simulink model "sampleModel1876"  (R2023a)
settings: Solver=VariableStepAuto  StartTime=0.0  StopTime=10.0  RelTol=1e-3
libraries: hdlsllib x5
settings Model: Creator=user1  LastModifiedBy=user1

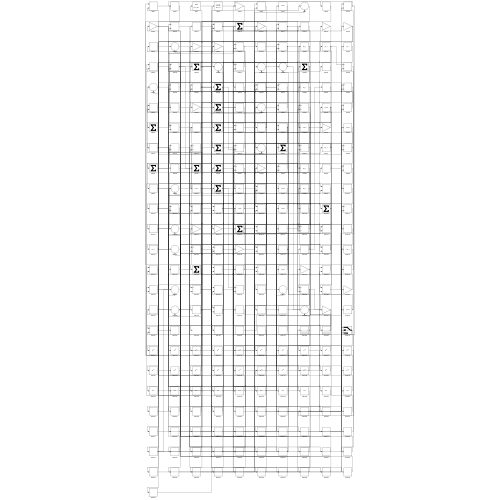
[thumbnail: Simulink's stored preview of the top-level diagram]
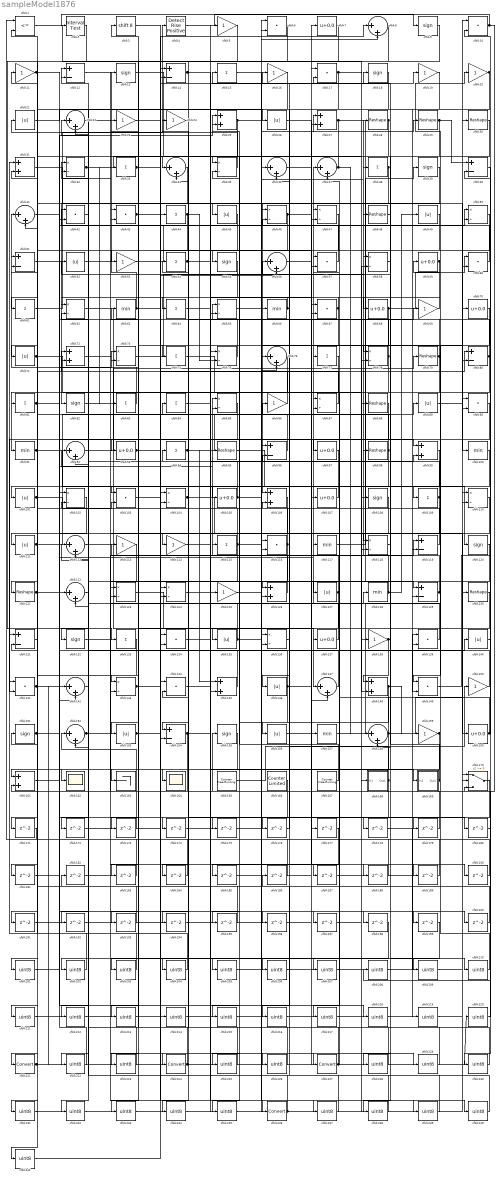
== system sampleModel1876 ==
  cfblk1 : RelationalOperator  Operator=<=  OutDataTypeStr=boolean  InputSameDT=off
  cfblk{6,10,17,42..43,57,60,67,90,103,116,134,139,141,144,149} (16 alike) : DotProduct  OutDataTypeStr=Inherit: Inherit via internal rule
  cfblk{63,66,91,100,117,128,157} (7 alike) : MinMax
  cfblk{21,26,45,49,52,71,89,101,111,127,135,140,146,153,156} (15 alike) : Abs  SaturateOnIntegerOverflow=off
  cfblk{32,35,46..47,50,58,62,65,73,75,78,85,87,102,104,110,118,123..124,136,143} (21 alike) : Product  Inputs=*/  RndMeth=Zero  SaturateOnIntegerOverflow=on
  cfblk{7,59,68,70,93,97,105,107,137,160} (10 alike) : Bias  Bias=0.0  SaturateOnIntegerOverflow=off
  cfblk{25,27,31,72,99,106,126,145,148,161} (10 alike) : Sum
  cfblk{9,13,18,39,55,82,108,120,132,151,155} (11 alike) : Signum
  cfblk{15,33,38,44,54,61,64,74,77,81,83..84,94,109,115,133} (16 alike) : Sum  Inputs=+
  cfblk{5,11,16,19..20,23..24,53,69,86,113..114,125,138,150,159} (16 alike) : Gain
  cfblk{8,22,34,36..37,41,56,76,92,112,122,142,147,152,158} (15 alike) : Sum  Inputs=|++
  cfblk{12,14,40,51,80,96,119,129,131,154} (10 alike) : Sum  Inputs=+-
  cfblk{28..30,48,79,88,95,98,121,130} (10 alike) : Reshape
  cfblk162 : Scope
  cfblk163 : Terminator
  cfblk164 : Scope
  cfblk165 : hdlsllib/Sources/Counter Free-Running  NumBits=16  tsamp=-1
  cfblk166 : hdlsllib/Sources/Counter Limited  uplimit=7  tsamp=-1
  cfblk167 : hdlsllib/Sources/Counter Free-Running  NumBits=16  tsamp=-1
  cfblk168 : Subsystem
      settings: LibrarySourceBlock=|
      | hdlsllib/Ports &
      | Subsystems/Subsystem
  cfblk169 : Subsystem
      settings: LibrarySourceBlock=|
      | hdlsllib/Ports &
      | Subsystems/Subsystem
  cfblk170 : Switch  SaturateOnIntegerOverflow=off  InputSameDT=off
  cfblk{171..200} (30 alike) : Delay  SampleTime=1
  cfblk2 : hdlsllib/Logic and Bit Operations/Interval Test  IntervalClosedRight=on  uplimit=0.5  IntervalClosedLeft=on  lowlimit=-0.5  OutDataTypeStr=boolean
  cfblk{201..220,222..223,225..226,228..235,237..241} (37 alike) : DataTypeConversion  OutDataTypeStr=uint8  SaturateOnIntegerOverflow=off  RndMeth=Floor
  cfblk{221,224,227,236} (4 alike) : DataTypeConversion  SaturateOnIntegerOverflow=off  RndMeth=Floor
  cfblk3 : ArithShift  BitShiftNumber=8
  cfblk4 : hdlsllib/Logic and Bit Operations/Detect Rise Positive  vinit=0  OutDataTypeStr=boolean
  wires:
  cfblk83/1 -> cfblk41/1
  cfblk47/1 -> cfblk153/1
  cfblk27/1 -> cfblk129/1, cfblk164/1, cfblk55/1
  cfblk2/1 -> cfblk133/1
  cfblk46/1 -> cfblk29/1, cfblk188/1, cfblk241/1
  cfblk94/1 -> cfblk145/1, cfblk58/2
  cfblk118/1 -> cfblk15/1
  cfblk38/1 -> cfblk106/1, cfblk121/1
  cfblk29/1 -> cfblk40/1, cfblk81/1, cfblk228/1
  cfblk157/1 -> cfblk20/1
  cfblk165/1 -> cfblk150/1
  cfblk95/1 -> cfblk120/1
  cfblk75/1 -> cfblk65/1
  cfblk111/1 -> cfblk89/1, cfblk119/2
  cfblk167/1 -> cfblk85/1
  cfblk39/1 -> cfblk82/1
  cfblk62/1 -> cfblk135/1
  cfblk132/1 -> cfblk128/1
  cfblk149/1 -> cfblk50/1
  cfblk63/1 -> cfblk13/1, cfblk127/1
  cfblk123/1 -> cfblk147/1
  cfblk30/1 -> cfblk61/1
  cfblk92/1 -> cfblk79/1
  cfblk117/1 -> cfblk39/1
  cfblk41/1 -> cfblk122/1
  cfblk69/1 -> cfblk66/1
  cfblk128/1 -> cfblk25/1, cfblk49/1
  cfblk112/1 -> cfblk224/1
  cfblk10/1 -> cfblk155/1, cfblk2/1
  cfblk16/1 -> cfblk71/1
  cfblk14/1 -> cfblk125/1, cfblk67/2
  cfblk137/1 -> cfblk37/1
  cfblk159/1 -> cfblk178/1, cfblk216/1
  cfblk78/1 -> cfblk126/1, cfblk54/1
  cfblk28/1 -> cfblk122/2, cfblk171/1
  cfblk168/1(Out1) -> cfblk106/2, cfblk234/1
  cfblk32/1 -> cfblk34/1, cfblk83/1
  cfblk96/1 -> cfblk11/1
  cfblk136/1 -> cfblk56/1
  cfblk57/1 -> cfblk3/1
  cfblk79/1 -> cfblk76/1, cfblk137/1, cfblk34/2
  cfblk17/1 -> cfblk111/1, cfblk80/2
  cfblk156/1 -> cfblk7/1
  cfblk126/1 -> cfblk85/2
  cfblk91/1 -> cfblk109/1, cfblk196/1
  cfblk80/1 -> cfblk132/1, cfblk35/2
  cfblk129/1 -> cfblk28/1, cfblk36/2
  cfblk119/1 -> cfblk94/1
  cfblk64/1 -> cfblk48/1
  cfblk51/1 -> cfblk33/1
  cfblk21/1 -> cfblk26/1
  cfblk20/1 -> cfblk96/1, cfblk149/2
  cfblk19/1 -> cfblk41/2
  cfblk106/1 -> cfblk145/2
  cfblk73/1 -> cfblk58/1
  cfblk25/1 -> cfblk47/2, cfblk194/1
  cfblk37/1 -> cfblk35/1, cfblk158/1
  cfblk53/1 -> cfblk47/1
  cfblk115/1 -> cfblk27/1, cfblk32/2, cfblk202/1
  cfblk135/1 -> cfblk12/1, cfblk8/2
  cfblk71/1 -> cfblk104/2, cfblk148/2
  cfblk146/1 -> cfblk32/1, cfblk180/1, cfblk235/1
  cfblk36/1 -> cfblk18/1
  cfblk61/1 -> cfblk4/1
  cfblk4/1 -> cfblk9/1
  cfblk88/1 -> cfblk141/2
  cfblk152/1 -> cfblk119/1, cfblk209/1
  cfblk48/1 -> cfblk68/1
  cfblk107/1 -> cfblk101/1
  cfblk116/1 -> cfblk31/2, cfblk173/1
  cfblk105/1 -> cfblk38/1, cfblk62/2
  cfblk50/1 -> cfblk143/1
  cfblk81/1 -> cfblk97/1, cfblk73/1
  cfblk142/1 -> cfblk152/2
  cfblk133/1 -> cfblk161/1
  cfblk43/1 -> cfblk44/1, cfblk50/2, cfblk56/2
  cfblk11/1 -> cfblk174/1, cfblk218/1
  cfblk143/1 -> cfblk14/1, cfblk80/1
  cfblk68/1 -> cfblk60/1, cfblk163/1
  cfblk138/1 -> cfblk148/1, cfblk98/1
  cfblk140/1 -> cfblk40/2
  cfblk153/1 -> cfblk8/1, cfblk190/1
  cfblk89/1 -> cfblk70/1
  cfblk160/1 -> cfblk115/1, cfblk10/2
  cfblk22/1 -> cfblk236/1
  cfblk60/1 -> cfblk43/1
  cfblk58/1 -> cfblk118/1
  cfblk9/1 -> cfblk53/1
  cfblk70/1 -> cfblk149/1
  cfblk158/1 -> cfblk42/1, cfblk30/1, cfblk191/1
  cfblk7/1 -> cfblk103/1
  cfblk150/1 -> cfblk57/1
  cfblk101/1 -> cfblk103/2, cfblk197/1
  cfblk42/1 -> cfblk12/2
  cfblk139/1 -> cfblk92/2
  cfblk13/1 -> cfblk108/1
  cfblk8/1 -> cfblk74/1
  cfblk102/1 -> cfblk221/1
  cfblk169/1(Out1) -> cfblk52/1, cfblk87/2
  cfblk109/1 -> cfblk24/1, cfblk154/2
  cfblk44/1 -> cfblk75/2, cfblk203/1
  cfblk144/1 -> cfblk77/1
  cfblk100/1 -> cfblk136/2
  cfblk55/1 -> cfblk123/2
  cfblk12/1 -> cfblk129/2
  cfblk35/1 -> cfblk21/1
  cfblk151/1 -> cfblk117/1, cfblk46/2
  cfblk77/1 -> cfblk146/1
  cfblk24/1 -> cfblk114/1
  cfblk125/1 -> cfblk87/1
  cfblk121/1 -> cfblk25/2, cfblk198/1
  cfblk145/1 -> cfblk63/1
  cfblk74/1 -> cfblk118/2
  cfblk87/1 -> cfblk72/1
  cfblk98/1 -> cfblk156/1, cfblk23/1
  cfblk66/1 -> cfblk16/1, cfblk64/1
  cfblk59/1 -> cfblk93/1, cfblk158/2
  cfblk1/1 -> cfblk88/1
  cfblk67/1 -> cfblk62/1, cfblk184/1, cfblk185/1, cfblk206/1
  cfblk104/1 -> cfblk160/1, cfblk99/2
  cfblk65/1 -> cfblk78/1
  cfblk122/1 -> cfblk162/1
  cfblk86/1 -> cfblk51/1
  cfblk52/1 -> cfblk116/2
  cfblk31/1 -> cfblk100/1
  cfblk33/1 -> cfblk57/2, cfblk45/1, cfblk19/1
  cfblk148/1 -> cfblk159/1, cfblk175/1, cfblk176/1
  cfblk154/1 -> cfblk161/2, cfblk17/2
  cfblk54/1 -> cfblk199/1, cfblk200/1
  cfblk56/1 -> cfblk157/1
  cfblk93/1 -> cfblk105/1, cfblk99/1, cfblk223/1
  cfblk108/1 -> cfblk143/2
  cfblk127/1 -> cfblk73/2, cfblk195/1
  cfblk141/1 -> cfblk69/1, cfblk95/1
  cfblk76/1 -> cfblk91/1
  cfblk45/1 -> cfblk154/1
  cfblk84/1 -> cfblk227/1
  cfblk147/1 -> cfblk86/1
  cfblk161/1 -> cfblk140/1
  cfblk114/1 -> cfblk169/1(In1)
  cfblk171/1 -> cfblk1/1
  cfblk18/1 -> cfblk172/1
  cfblk172/1 -> cfblk104/1
  cfblk173/1 -> cfblk152/1
  cfblk174/1 -> cfblk76/2
  cfblk175/1 -> cfblk126/2
  cfblk176/1 -> cfblk96/2
  cfblk103/1 -> cfblk179/1
  cfblk179/1 -> cfblk123/1
  cfblk155/1 -> cfblk181/1
  cfblk181/1 -> cfblk142/2
  cfblk34/1 -> cfblk183/1
  cfblk183/1 -> cfblk141/1
  cfblk184/1 -> cfblk31/1
  cfblk185/1 -> cfblk147/2
  cfblk186/1 -> cfblk43/2
  cfblk82/1 -> cfblk187/1
  cfblk187/1 -> cfblk139/1
  cfblk188/1 -> cfblk75/1
  cfblk26/1 -> cfblk189/1
  cfblk189/1 -> cfblk136/1
  cfblk190/1 -> cfblk46/1
  cfblk191/1 -> cfblk67/1
  cfblk113/1 -> cfblk192/1
  cfblk192/1 -> cfblk14/2
  cfblk97/1 -> cfblk193/1
  cfblk193/1 -> cfblk92/1
  cfblk194/1 -> cfblk65/2
  cfblk195/1 -> cfblk51/2
  cfblk196/1 -> cfblk27/2
  cfblk197/1 -> cfblk78/2
  cfblk200/1 -> cfblk1/2
  cfblk131/1 -> cfblk201/1
  cfblk201/1 -> cfblk42/2
  cfblk202/1 -> cfblk131/1
  cfblk203/1 -> cfblk131/2
  cfblk90/1 -> cfblk204/1
  cfblk204/1 -> cfblk151/1
  cfblk166/1 -> cfblk205/1
  cfblk205/1 -> cfblk90/1
  cfblk206/1 -> cfblk90/2
  cfblk110/1 -> cfblk207/1
  cfblk207/1 -> cfblk139/2
  cfblk180/1 -> cfblk208/1
  cfblk208/1 -> cfblk110/1
  cfblk209/1 -> cfblk110/2
  cfblk134/1 -> cfblk210/1
  cfblk210/1 -> cfblk59/1
  cfblk85/1 -> cfblk211/1
  cfblk211/1 -> cfblk134/1
  cfblk198/1 -> cfblk212/1
  cfblk212/1 -> cfblk134/2
  cfblk130/1 -> cfblk213/1
  cfblk213/1 -> cfblk17/1
  cfblk23/1 -> cfblk214/1
  cfblk214/1 -> cfblk130/1
  cfblk177/1 -> cfblk215/1
  cfblk215/1 -> cfblk116/1
  cfblk216/1 -> cfblk177/1
  cfblk170/1 -> cfblk217/1
  cfblk217/1 -> cfblk138/1
  cfblk218/1 -> cfblk170/1
  cfblk178/1 -> cfblk219/1
  cfblk219/1 -> cfblk170/2
  cfblk220/1 -> cfblk170/3
  cfblk221/1 -> cfblk220/1, cfblk107/1, cfblk142/1
  cfblk99/1 -> cfblk222/1
  cfblk222/1 -> cfblk102/1
  cfblk223/1 -> cfblk102/2
  cfblk224/1 -> cfblk36/1, cfblk144/1
  cfblk49/1 -> cfblk225/1
  cfblk225/1 -> cfblk112/1
  cfblk72/1 -> cfblk226/1
  cfblk226/1 -> cfblk112/2
  cfblk227/1 -> cfblk113/1, cfblk37/2
  cfblk228/1 -> cfblk84/1
  cfblk182/1 -> cfblk229/1
  cfblk229/1 -> cfblk144/2
  cfblk40/1 -> cfblk230/1
  cfblk230/1 -> cfblk182/1
  cfblk5/1 -> cfblk231/1
  cfblk231/1 -> cfblk168/1(In1)
  cfblk120/1 -> cfblk232/1
  cfblk232/1 -> cfblk5/1
  cfblk6/1 -> cfblk233/1
  cfblk233/1 -> cfblk10/1
  cfblk234/1 -> cfblk6/1
  cfblk235/1 -> cfblk6/2
  cfblk236/1 -> cfblk72/2, cfblk60/2
  cfblk3/1 -> cfblk237/1
  cfblk237/1 -> cfblk22/1
  cfblk199/1 -> cfblk238/1
  cfblk238/1 -> cfblk22/2
  cfblk124/1 -> cfblk239/1
  cfblk239/1 -> cfblk186/1
  cfblk15/1 -> cfblk240/1
  cfblk240/1 -> cfblk124/1
  cfblk241/1 -> cfblk124/2

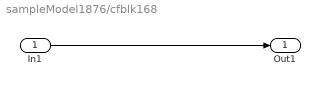
== system sampleModel1876/cfblk168 ==
  In1 : Inport
  Out1 : Outport
  wires:
  In1/1 -> Out1/1

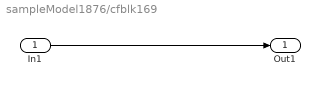
== system sampleModel1876/cfblk169 ==
  In1 : Inport
  Out1 : Outport
  wires:
  In1/1 -> Out1/1
